simulink library "UserBlocks"  (R2014a)
settings: Solver=ode45  SolverMode=SingleTasking  StartTime=0.0  StopTime=10.0  RelTol=1e-3
values from neighbouring files (symbols this model uses):
  a = param.a    [DSC_Control_Analysis.m]    (also in DSC_Control_Analysis_Exp.m; DSC_Speed_Control_Analysis.m; EmpiricalTireCurves.m = 1.35; FFW_Fx.m = sqrt(curvature/(2*clothoidLength)))
  b = 1.15    [EmpiricalTireCurves.m]
  Cfls = Cfl    [EC_params_nissan.m]
  Crls = Crl    [EC_params_nissan.m]
  d0 = CSTR.d0    [Ext_MPCPara.m]
  freq = Fs/2*linspace(0,1,NFFT/2)    [AACplottingcode.m]    (also in If_alpha_tp_observer.m; If_alpha_tp_observer_for_c_code.m; If_alpha_tp_observer_shoreline.m)
  Iz = param.Iz    [DSC_Control_Analysis.m]    (also in DSC_Control_Analysis_Exp.m; DSC_Speed_Control_Analysis.m; EmpiricalTireCurves.m = 1300)
  K = 10    [EC_params_nissan.m]
  Ks = -10    [EC_params_nissan.m]
  Ksl = -10    [EC_params_nissan.m]
  Kt = 40000    [EC_params_nissan.m]
  Ku = -40000    [EC_params_nissan.m]
  m = 1724    [EmpiricalTireCurves.m]
  mu_s = mu_p    (= 0.6)    [EC_params_nissan.m]    (also in EmpiricalTireCurves.m = 0.55)
  Ns = 10    [EC_params_nissan.m]
  num = num+MTnum(m)    [Build_MtMuMy.m]
  q = 1    [EC_params_nissan.m]
  Taoh = CSTR.Taoh    [Ext_MPCPara.m]
  Ts = 0.002    [DSC_Control_Analysis.m]    (also in DSC_Control_Analysis_Exp.m; DSC_Speed_Control_Analysis.m; EC_params_nissan.m; Ext_MPCPara.m = SSD.Ts)
undefined symbols (not defined in the file or in its folder): acceAmp, ack, alphaFrontSteeringLimit, alphaFrontTable, bit, c, Cfl, Crl, CSTR, dden, deltaPsiDotGain, deltDist, den, denafilt, dnum, elaDotGain, filtera, filterb, frontAlphaLookup, frontForceLookup, FuelStartCalTime, FyFtable, gpsins, h, h_roll, hal_filter_den, hal_filter_num, hwx, hwy5, initAcce, initSpeed, isDriverNoise, lkparams, mapDataFull, mapMatchingParams, maxFrontForce, maxNumSegs, mdPtrs, numafilt, param, rearAlphaLookup, rfl, rfr, rrl, rrr, sglu, SIMP, simuCond, slimFxl, slimFxu, sliml, slimMll, slimMlr, slimMul, slimMur, slimu, sr, SSD, Standard, steering_limit ... (+7)
libraries: simulink x28, slrtlib x18, UserBlocks x6, slrtsoftinglib x6, MickLibBlocks x1, DriftControllerLibrary x1
(part 2 of 6)

== system UserBlocks/Diagnostic System/Filtering ==
  Residuals : Inport
  Another low-pass filter : Subsystem
      mask init:
      | %[num,den]=ellip(4,1,100,.01);
      | num=1e-4*[0.10928026599394  -0.39276857908969   0.56935540895543  -0.39276857908970   0.10928026599394];
      | den=[1  -3.96909955856226   5.90874845132499  -3.91017494417814   0.97052631831922];
  Bus Creator : BusCreator  Inputs=8
  Bus Selector : BusSelector  OutputSignals=Resistance,Motor Constant,Lsa,Rsa,yr,Gearbox Angle,Steering Angle,Current Error
  Low-pass filter : Subsystem
      mask init:
      | %[num,den]=ellip(4,1,100,.1);
      | num=1e-3*[0.23296035547458   0.49053981729288   0.64935382394602   0.49053981729287   0.23296035547457];
      | den=[1  -3.60782459052443   4.97952457348602  -3.11098657182084   0.74163873692417];
  Filtered Residuals : Outport
  wires:
  Residuals/1 -> Bus Selector/1
  Bus Selector/7 -> Bus Creator/7  "<Steering Angle>"
  Bus Selector/1 -> Bus Creator/1  "<Resistance>"
  Bus Selector/2 -> Bus Creator/2  "<Motor Constant>"
  Bus Selector/3 -> Bus Creator/3  "<Lsa>"
  Bus Selector/4 -> Bus Creator/4  "<Rsa>"
  Bus Selector/5 -> Bus Creator/5  "<yr>"
  Bus Selector/6 -> Low-pass filter/1(In1)  "<Gearbox Angle>"
  Bus Creator/1 -> Filtered Residuals/1
  Bus Selector/8 -> Another low-pass filter/1(In1)  "<Current Error>"
  Another low-pass filter/1(Out1) -> Bus Creator/8  "Filtered Current Error"
  Low-pass filter/1(Out1) -> Bus Creator/6  "Filtered Gearbox Angle"

== system UserBlocks/Diagnostic System/Isolation ==
  Boolean Residuals : Inport
  Fcn : Fcn  Expr=u[1]+2*u[2]+4*u[3]+8*u[4]+16*u[5]+32*u[6]+64*u[7]+128*u[8]+256*u[9]+512*u[10]+1024*u[11]+2048*u[12]+4096*u[13]
  Diagnosis : Outport
  wires:
  Boolean Residuals/1 -> Fcn/1
  Fcn/1 -> Diagnosis/1

== system UserBlocks/Diagnostic System/Residual Generation ==
  Steering Motors : Inport
  INS : Inport  Port=2
  Wheelspeeds : Inport  Port=3
  Current Commands : Inport  Port=4
  Handwheel : Inport  Port=5
  Roll Angle : Inport  Port=6
  Amplifier Model : Subsystem
      mask init:
      | p1_params
  Average : Gain  Gain=.5*[ 1 1]  Multiplication=Matrix(K*u)  SaturateOnIntegerOverflow=on  OutDataTypeStr=Inherit: Same as input  ParamDataTypeStr=Inherit: Same as input
  Bus Creator : BusCreator  Inputs=11
  Controller Model : Subsystem
      mask init:
      | p1_params
      | SteeringController
  Gearbox Model : Subsystem
      mask init:
      | p1_params
  Ground{,1..5} (6 alike) : Ground
  Jihan!!! : Gain  Gain=pi/180  SaturateOnIntegerOverflow=on  OutDataTypeStr=Inherit: Same as input  ParamDataTypeStr=Inherit: Same as input
  Motor Parameter Estimators : Subsystem
      mask init:
      | p1_params
      | InitMotorEstimator
  Select: Yaw Rate : Subsystem  mask{indices=1, width=6}
      mask prompts: indices "Signal indices"; width "Input width"
      mask init:
      | ic=length(indices);
      | 
      | K=zeros(ic,width);
      | 
      | for ii=1:ic,
      | 	K(ii,indices(ii))=1;
      | end
      mask Display: disp(indices)
  Terminator{,1..4} (5 alike) : Terminator
  Residuals : Outport
  wires:
  Steering Motors/1 -> Motor Parameter Estimators/1(Steering Motors), Gearbox Model/1("Steering Motors "), Controller Model/1("Steering Motors "), Amplifier Model/1("Steering Motors "), Terminator/1
  Motor Parameter Estimators/1(Resistances) -> Bus Creator/1  "Resistance"
  Motor Parameter Estimators/2(Motor Constants) -> Bus Creator/2  "Motor Constant"
  Bus Creator/1 -> Residuals/1
  Current Commands/1 -> Motor Parameter Estimators/2(Current Commands), Amplifier Model/2(Current Commands), Terminator2/1
  Select: Yaw Rate/1(Out1) -> Terminator1/1
  INS/1 -> Select: Yaw Rate/1(In1)
  Average/1 -> Terminator3/1
  Wheelspeeds/1 -> Average/1
  Gearbox Model/1(A) -> Bus Creator/9  "Gearbox Angle"
  Controller Model/1(B) -> Bus Creator/10  "Steering Angle"
  Handwheel/1 -> Controller Model/2(Handwheel)
  Amplifier Model/1(B) -> Bus Creator/11  "Current Error"
  Roll Angle/1 -> Jihan!!!/1
  Jihan!!!/1 -> Terminator4/1
  Ground/1 -> Bus Creator/3  "Yaw Rate A"
  Ground1/1 -> Bus Creator/4  "Yaw Rate B"
  Ground2/1 -> Bus Creator/5  "Yaw Rate C"
  Ground3/1 -> Bus Creator/6  "Lsa"
  Ground4/1 -> Bus Creator/7  "Rsa"
  Ground5/1 -> Bus Creator/8  "yr"

== system UserBlocks/EnvEnv Connection/Ackermann Correction ==
  Ackermann Angle : Inport
  left ackermann ideal correction angle : Fcn  Expr=u/(1-u*ack*param.tw/2/(param.a+param.b))
  right ackermann ideal correction angle : Fcn  Expr=u/(1+u*ack*param.tw/2/(param.a+param.b))
  L Steer Angle : Outport
  R Steer Angle : Outport  Port=2
  wires:
  Ackermann Angle/1 -> right ackermann ideal correction angle/1, left ackermann ideal correction angle/1
  right ackermann ideal correction angle/1 -> R Steer Angle/1
  left ackermann ideal correction angle/1 -> L Steer Angle/1

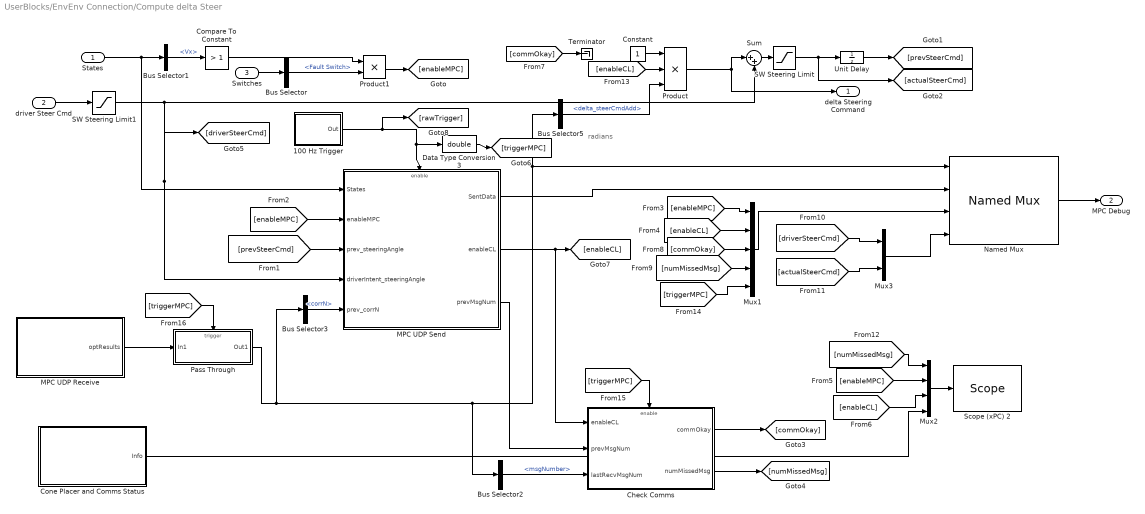
== system UserBlocks/EnvEnv Connection/Compute delta Steer ==
  note: radians
  States : Inport
  driver Steer Cmd : Inport  Port=2
  Switches : Inport  Port=3
  100 Hz Trigger : Subsystem
  Bus Selector : BusSelector  OutputSignals=Fault Switch
  Bus Selector1 : BusSelector  OutputSignals=Vx
  Bus Selector2 : BusSelector  OutputSignals=msgNumber
  Bus Selector3 : BusSelector  OutputSignals=corrN
  Bus Selector5 : BusSelector  OutputSignals=delta_steerCmdAdd
  Check Comms : Subsystem  TreatAsAtomicUnit=on
  Compare To Constant : simulink/Logic and Bit Operations/Compare To Constant  relop=>  const=1  OutDataTypeStr=uint8  ZeroCross=off
  Cone Placer and Comms Status : Subsystem
  Constant : Constant
  Data Type Conversion3 : DataTypeConversion  OutDataTypeStr=double
  MPC UDP Receive : Subsystem
  MPC UDP Send : Subsystem
  Mux1 : Mux  Inputs=5
  Mux2 : Mux
  Mux3 : Mux  Inputs=2
  Named Mux : UserBlocks/MPC CAN Connection/Named Mux  fname=datadescEnvEnv
  Pass Through : Subsystem  TreatAsAtomicUnit=on
  Product : Product  Inputs=3  RndMeth=Zero
  Product1 : Product  RndMeth=Zero
  SW Steering Limit : Saturate  UpperLimit=steering_limit*pi/180  LowerLimit=-steering_limit*pi/180
  SW Steering Limit1 : Saturate  UpperLimit=steering_limit*pi/180  LowerLimit=-steering_limit*pi/180
  Scope (xPC) 2 : slrtlib/Displays and Logging/Scope   scopeno=2  scopetype=Target  autostart=on  viewmode=Numerical  formatstr="' Missed Msgs:   %6.0f, EnableMPC:    %1.0f, EnableCL:     %1.0f, Bumper E Pos [m]:    %4.2f, Bumper N Pos [m]:    %4.2f, Num Laptop Msgs: %5.0f, Num Veh Msgs:    %5.0f'"  grid=on  ylimits=[0,0]  nosamples=round(1/Ts)/20  noprepostsamples=0  interleave=1  triggermode=FreeRun  triggersignal=1  trigsignalfromport=off  triggerlevel=0.0  triggerslope=Either  triggerscope=1  triggersample=0  filename=data.dat  mode=Lazy  writesize=512  autorestart=off  dynamicfilemode=off  maxwritefilesize=512*1024^2
  Sum : Sum  Inputs=|++
  Terminator : Terminator
  Unit Delay : UnitDelay  SampleTime=-1
  delta Steering Command : Outport
  MPC Debug : Outport  Port=2
  wires:
  Cone Placer and Comms Status/1(Info) -> Mux2/4
  [numMissedMsg] -> Mux2/1
  [enableCL] -> Mux2/3
  [enableMPC] -> Mux2/2
  Mux2/1 -> Scope (xPC) 2/1
  Bus Selector3/1 -> MPC UDP Send/5(prev_corrN)  "<corrN>"
  [triggerMPC] -> Pass Through/Trigger
  MPC UDP Receive/1(optResults) -> Pass Through/1(In1)
  MPC UDP Send/3(prevMsgNum) -> Check Comms/2(prevMsgNum)
  Bus Selector2/1 -> Check Comms/3(lastRecvMsgNum)  "<msgNumber>"
  [triggerMPC] -> Check Comms/Enable
  Check Comms/2(numMissedMsg) -> [numMissedMsg]
  Check Comms/1(commOkay) -> [commOkay]
  Data Type Conversion3/1 -> [triggerMPC]
  [triggerMPC] -> Mux1/5
  Pass Through/1(Out1) -> Bus Selector3/1, Bus Selector5/1, Named Mux/1, Bus Selector2/1
  Mux1/1 -> Named Mux/3
  Constant/1 -> Product/1
  [commOkay] -> Terminator/1
  [enableCL] -> Product/2
  MPC UDP Send/2(enableCL) -> Check Comms/1(enableCL), [enableCL]
  [enableMPC] -> MPC UDP Send/2(enableMPC)
  100 Hz Trigger/1(Out) -> [rawTrigger], Data Type Conversion3/1, MPC UDP Send/Enable
  Sum/1 -> SW Steering Limit/1
  Unit Delay/1 -> [prevSteerCmd]
  SW Steering Limit/1 -> [actualSteerCmd], Unit Delay/1
  driver Steer Cmd/1 -> SW Steering Limit1/1
  [actualSteerCmd] -> Mux3/2
  [driverSteerCmd] -> Mux3/1
  Mux3/1 -> Named Mux/4
  SW Steering Limit1/1 -> [driverSteerCmd], MPC UDP Send/4(driverIntent_steeringAngle), Sum/2
  [numMissedMsg] -> Mux1/4
  [commOkay] -> Mux1/3
  Product/1 -> delta Steering Command/1, Sum/1
  [enableCL] -> Mux1/2
  [enableMPC] -> Mux1/1
  MPC UDP Send/1(SentData) -> Named Mux/2
  [prevSteerCmd] -> MPC UDP Send/3(prev_steeringAngle)
  Named Mux/1 -> MPC Debug/1
  Bus Selector5/1 -> Product/3  "<delta_steerCmdAdd>"
  Bus Selector1/1 -> Compare To Constant/1  "<Vx>"
  States/1 -> MPC UDP Send/1(States), Bus Selector1/1
  Switches/1 -> Bus Selector/1
  Bus Selector/1 -> Product1/2  "<Fault Switch>"
  Compare To Constant/1 -> Product1/1
  Product1/1 -> [enableMPC]

== system UserBlocks/EnvEnv Connection/Subsystem ==
  Handwheel : Inport
  Switches : Inport  Port=2
  Bus Selector2 : BusSelector  OutputSignals=Primary
  Bus Selector4 : BusSelector  OutputSignals=Auto-Steer Switch
  HAL-9000 : UserBlocks/Steering Controller/HAL-9000  enabled=on  maneuver=Step  amplitude=12/sr  delay=1  duration=10  startfreq=.7  endfreq=.7
  Heavy Filter : DiscreteFilter  Numerator=hal_filter_num  Denominator=hal_filter_den  SampleTime=Ts
  Nominal Filter : DiscreteFilter  Numerator=[10*2*pi*Ts]  Denominator=[1 10*2*pi*Ts-1]  SampleTime=Ts
  Steering Ratio : Gain  Gain=1/10  SaturateOnIntegerOverflow=on  OutDataTypeStr=Inherit: Same as input  ParamDataTypeStr=Inherit: Same as input
  Steering Ratio1 : Gain  Gain=1/10  SaturateOnIntegerOverflow=on  OutDataTypeStr=Inherit: Same as input  ParamDataTypeStr=Inherit: Same as input
  Sum1 : Sum  Inputs=++|
  Switch : Switch  Threshold=0.5
  Steering Output : Outport
  wires:
  Switch/1 -> Steering Output/1
  Sum1/1 -> Switch/1
  HAL-9000/1 -> Sum1/2
  Steering Ratio1/1 -> Sum1/1
  Steering Ratio/1 -> Switch/3
  Switches/1 -> Bus Selector4/1
  Bus Selector4/1 -> Switch/2, HAL-9000/1  "<Auto-Steer Switch>"
  Heavy Filter/1 -> Steering Ratio1/1
  Bus Selector2/1 -> Heavy Filter/1, Nominal Filter/1  "<Primary>"
  Nominal Filter/1 -> Steering Ratio/1
  Handwheel/1 -> Bus Selector2/1

== system UserBlocks/Envelope control with Differential drive/acc_noise_cut_filter ==
  In1 : Inport
  Butterworth Filter : DiscreteFilter  Numerator=numafilt  Denominator=denafilt  SampleTime=0.002
  Out1 : Outport
  wires:
  In1/1 -> Butterworth Filter/1
  Butterworth Filter/1 -> Out1/1

== system UserBlocks/Envelope control with Differential drive/acc_noise_cut_filter1 ==
  In1 : Inport
  Butterworth Filter : DiscreteFilter  Numerator=numafilt  Denominator=denafilt  SampleTime=0.002
  Out1 : Outport
  wires:
  Butterworth Filter/1 -> Out1/1
  In1/1 -> Butterworth Filter/1

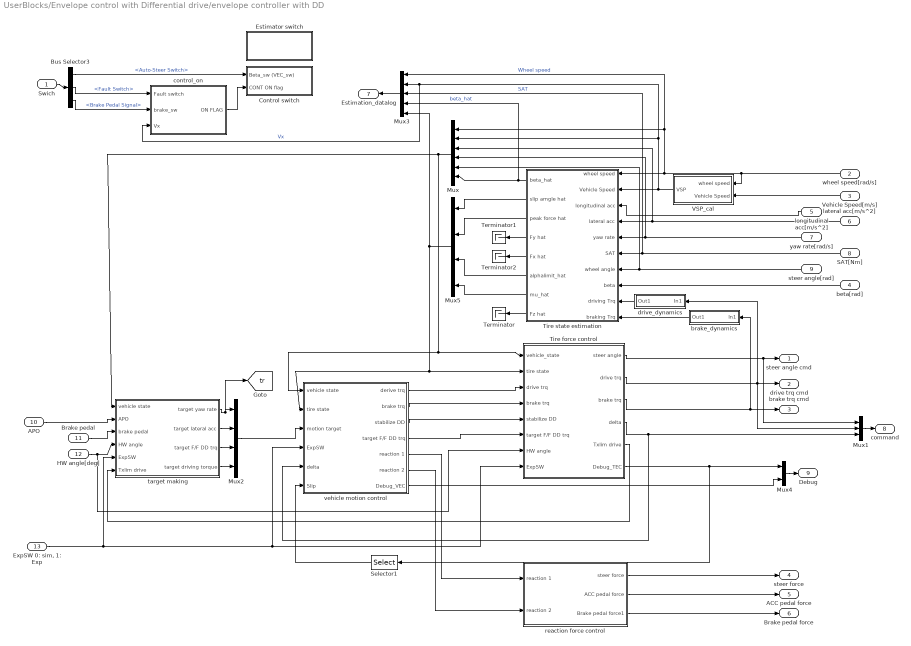
== system UserBlocks/Envelope control with Differential drive/envelope controller with DD ==
  Swich : Inport
  wheel speed[rad/s] : Inport  Port=2
  Vehicle Speed[m/s] : Inport  Port=3
  beta[rad] : Inport  Port=4
  longitudinal acc[m/s^2] : Inport  Port=5
  lateral acc[m/s^2] : Inport  Port=6
  yaw rate[rad/s] : Inport  Port=7
  SAT[Nm] : Inport  Port=8
  steer angle[rad] : Inport  Port=9
  APO : Inport  Port=10
  Brake pedal : Inport  Port=11
  HW angle[deg] : Inport  Port=12
  "ExpSW 0: sim, 1: Exp" : Inport  Port=13
  Bus Selector3 : BusSelector  OutputSignals=Auto-Steer Switch,Fault Switch,Brake Pedal Signal
  Control switch : Subsystem
  Estimator switch : Subsystem
  Mux : Mux  Inputs=6
  Mux1 : Mux  Inputs=3
  Mux2 : Mux
  Mux3 : Mux  Inputs=5
  Mux4 : Mux  Inputs=2
  Mux5 : Mux
  Selector1 : Selector  InputPortWidth=8  Indices=[5:6]
  Terminator : Terminator
  Terminator1 : Terminator
  Terminator2 : Terminator
  Tire force control : Subsystem
      mask init:
      | p1_params
      | EC_params_nissan
      | load slimmap
      | [filterb,filtera]=butter(2,0.03);
  Tire state estimation : Subsystem
      mask init:
      | p1_params
      | EC_params_nissan
  VSP_cal : Subsystem
      mask init:
      | p1_params
      | EC_params_nissan
  brake_dynamics : Subsystem
  control_on : Subsystem
  drive_dynamics : Subsystem
  reaction force control : Subsystem
  target making : Subsystem
      mask init:
      | p1_params
      | EC_params_nissan
      | % FFDDmodel_cal
      | [dnum,dden]=c2dm([1 0],[0.1 1],0.002,'tustin');
  vehicle motion control : Subsystem
      mask init:
      | p1_params
      | EC_params_nissan
      | load stableareamap.mat
  steer angle cmd : Outport
  drive trq cmd : Outport  Port=2
  brake trq cmd : Outport  Port=3
  steer force : Outport  Port=4
  ACC pedal force : Outport  Port=5
  Brake pedal force : Outport  Port=6
  Estimation_datalog : Outport  Port=7
  command : Outport  Port=8
  Debug : Outport  Port=9
  tag scope: tr=global
  wires:
  vehicle motion control/4(target F/F DD trq) -> Tire force control/6(target F/F DD trq)
  Selector1/1 -> vehicle motion control/6(Slip)
  Tire force control/5(Txlim drive) -> target making/6(Txlim drive)
  target making/4(target driving torque) -> Mux2/4
  lateral acc[m/s^2]/1 -> Mux/3, Tire state estimation/4(lateral acc)
  yaw rate[rad/s]/1 -> Mux/4, Tire state estimation/5(yaw rate)
  HW angle[deg]/1 -> target making/4(HW angle), Tire force control/7(HW angle)
  APO/1 -> target making/2(APO)
  Brake pedal/1 -> target making/3(brake pedal)
  target making/2(target lateral acc) -> Mux2/2
  target making/3(target F/F DD trq) -> Mux2/3
  Mux2/1 -> vehicle motion control/3(motion target)
  Tire force control/1(steer angle) -> steer angle cmd/1, Mux1/1
  Tire force control/2(drive trq) -> drive trq cmd/1, drive_dynamics/1(In1), Mux1/2
  Tire force control/3(brake trq) -> brake trq cmd/1, brake_dynamics/1(In1)
  vehicle motion control/1(derive trq) -> Tire force control/3("drive trq ")
  vehicle motion control/2(brake trq) -> Tire force control/4("brake trq ")
  vehicle motion control/5(reaction 1) -> reaction force control/1(reaction 1)
  vehicle motion control/6(reaction 2) -> reaction force control/2(reaction 2)
  reaction force control/1(steer force) -> steer force/1
  reaction force control/2(ACC pedal force) -> ACC pedal force/1
  reaction force control/3(Brake pedal force1) -> Brake pedal force/1
  wheel speed[rad/s]/1 -> Mux/1, Mux3/1, Tire state estimation/1(wheel speed), VSP_cal/1(wheel speed)  "Wheel speed"
  SAT[Nm]/1 -> Mux3/3, Tire state estimation/6(SAT)  "SAT"
  Tire state estimation/2(slip amgle hat) -> Mux5/1
  Tire state estimation/3(peak force hat) -> Mux5/2
  Tire state estimation/8(Fz hat) -> Terminator/1
  Mux3/1 -> Estimation_datalog/1
  vehicle motion control/3(stabilize DD) -> Tire force control/5(stabilize DD)
  Mux/1 -> vehicle motion control/1(vehicle state), Tire force control/1(vehicle_state), target making/1(vehicle state)
  Mux5/1 -> vehicle motion control/2(tire state), Tire force control/2(tire state), Mux3/5
  drive_dynamics/1(Out1) -> Tire state estimation/9(driving Trq)
  brake_dynamics/1(Out1) -> Tire state estimation/10(braking Trq)
  steer angle[rad]/1 -> Mux/5, Tire state estimation/7(wheel angle)
  Tire force control/4(delta) -> vehicle motion control/5(delta), Mux1/3
  target making/1(target yaw rate) -> Mux2/1, [tr]
  beta[rad]/1 -> Tire state estimation/8(beta)
  Tire state estimation/1(beta_hat) -> Mux/6, Mux3/4  "beta_hat"
  VSP_cal/1(VSP) -> control_on/3(Vx), Mux3/2, Mux/2, Tire state estimation/2(Vehicle Speed)  "Vx"
  Vehicle Speed[m/s]/1 -> VSP_cal/2(Vehicle Speed)
  Mux1/1 -> command/1
  Tire state estimation/4(Fy hat) -> Terminator1/1
  Tire state estimation/5(Fx hat) -> Terminator2/1
  Tire state estimation/7(mu_hat) -> Mux5/4
  Tire state estimation/6(alphalimit_hat) -> Mux5/3
  Tire force control/6(Debug_TEC) -> Selector1/1, Mux4/1
  vehicle motion control/7(Debug_VEC) -> Mux4/2
  Mux4/1 -> Debug/1
  "ExpSW 0: sim, 1: Exp"/1 -> target making/5(ExpSW), vehicle motion control/4(ExpSW), Tire force control/8(ExpSW)
  longitudinal acc[m/s^2]/1 -> Tire state estimation/3(longitudinal acc)
  control_on/1(ON FLAG) -> Control switch/2(CONT ON flag)
  Swich/1 -> Bus Selector3/1
  Bus Selector3/2 -> control_on/1(Fault switch)  "<Fault Switch>"
  Bus Selector3/3 -> control_on/2(brake_sw)  "<Brake Pedal Signal>"
  Bus Selector3/1 -> Control switch/1(Beta_sw (VEC_sw))  "<Auto-Steer Switch>"

== system UserBlocks/Envelope control with Differential drive/wheel_speed_dynamics ==
  In1 : Inport
  Butterworth Filter{,1..3} (4 alike) : DiscreteFilter  Numerator=filterb  Denominator=filtera  SampleTime=0.002
  Demux : Demux
  Mux : Mux
  rev/s to rad/s : Gain  Gain=2*pi
  ticks/sample to rev/s : Gain  Gain="1/(48*2)  *  1/Ts"
  Out1 : Outport
  wires:
  Demux/4 -> Butterworth Filter2/1
  Demux/3 -> Butterworth Filter3/1
  Demux/2 -> Butterworth Filter/1
  Demux/1 -> Butterworth Filter1/1
  Mux/1 -> Out1/1
  Butterworth Filter/1 -> Mux/1
  Butterworth Filter1/1 -> Mux/2
  Butterworth Filter2/1 -> Mux/3
  Butterworth Filter3/1 -> Mux/4
  ticks/sample to rev/s/1 -> rev/s to rad/s/1
  rev/s to rad/s/1 -> Demux/1
  In1/1 -> ticks/sample to rev/s/1

== system UserBlocks/LQACC/PIDACC ==
  Switches : Inport
  Vehicle States : Inport  Port=2
  Go Pedal1 : Inport  Port=3
  Bus Creator : BusCreator  Inputs=2
  Bus Selector : BusSelector  OutputSignals=Vx,axCG
  Bus Selector1 : BusSelector  OutputSignals=Fault Switch
  Car-Following System : Subsystem
  Demux : Demux  Outputs=3
  Discrete Filter : DiscreteFilter  Numerator=[0.006]  Denominator=[1.006 -1]  SampleTime=0.002
  MPC MTCACC : Subsystem
  PreVehicle : Subsystem
  Selection : Constant  Value=simuCond
  Subsystem : Subsystem
  Switch1 : Switch  Criteria=u2 > Threshold  Threshold=0.5
  FxCommands(N) : Outport
  PreAcce(m/s2) : Outport  Port=2
  PreSpeec(m/s) : Outport  Port=3
  epsilon : Outport  Port=4
  DesDist(m) : Outport  Port=5
  ActDist(m) : Outport  Port=6
  desAcce(m/s2) : Outport  Port=7
  distErr : Outport  Port=8
  relVEL : Outport  Port=9
  vehACCE : Outport  Port=10
  wires:
  Discrete Filter/1 -> Subsystem/1(ax), desAcce(m/s2)/1
  MPC MTCACC/2(desAcce) -> Discrete Filter/1
  Demux/3 -> vehACCE/1
  Demux/2 -> relVEL/1
  Demux/1 -> distErr/1
  Subsystem/1(Volt(V)1) -> Switch1/1
  Bus Selector/2 -> Car-Following System/4(vehAcce)  "<axCG>"
  Bus Selector/1 -> Car-Following System/3(vehSpd)  "<Vx>"
  Car-Following System/5(DesDist) -> DesDist(m)/1
  MPC MTCACC/1(epsilon) -> epsilon/1
  Car-Following System/3(actDist) -> MPC MTCACC/3(actDist), ActDist(m)/1
  Car-Following System/2(PV_acce) -> MPC MTCACC/2(PreAcce)
  Car-Following System/4(VehSpd) -> MPC MTCACC/4(vehSpd)
  PreVehicle/2(PreSpeed) -> Car-Following System/2(PVvel), PreSpeec(m/s)/1
  PreVehicle/1(PreAcce) -> Car-Following System/1(PVacce), PreAcce(m/s2)/1
  Selection/1 -> PreVehicle/1(Pattern)
  Car-Following System/1(SysOut) -> Demux/1, MPC MTCACC/1(SysOut)
  Switches/1 -> Bus Selector1/1
  Vehicle States/1 -> Bus Selector/1
  Bus Selector1/1 -> Switch1/2  "<Fault Switch>"
  Switch1/1 -> Bus Creator/1, Bus Creator/2
  Bus Creator/1 -> FxCommands(N)/1
  Go Pedal1/1 -> Switch1/3

== system UserBlocks/MPC CAN Connection/Ackermann Correction ==
  Ackermann Angle : Inport
  left ackermann ideal correction angle : Fcn  Expr=u/(1-u*ack*param.tw/2/(param.a+param.b))
  right ackermann ideal correction angle : Fcn  Expr=u/(1+u*ack*param.tw/2/(param.a+param.b))
  L Steer Angle : Outport
  R Steer Angle : Outport  Port=2
  wires:
  left ackermann ideal correction angle/1 -> L Steer Angle/1
  right ackermann ideal correction angle/1 -> R Steer Angle/1
  Ackermann Angle/1 -> left ackermann ideal correction angle/1, right ackermann ideal correction angle/1

== system UserBlocks/MPC CAN Connection/Force Feedback ==
  MPC Addition : Inport
  Feedback gain : Gain  Gain=steer_gain
  Saturation1 : Saturate  UpperLimit=current_limit  LowerLimit=-current_limit
  FFB Current : Outport
  wires:
  Feedback gain/1 -> Saturation1/1
  MPC Addition/1 -> Feedback gain/1
  Saturation1/1 -> FFB Current/1

== system UserBlocks/MPC CAN Connection/MPC CAN Receive ==
  "CAN bit-unpacking " : slrtlib/CAN/Utilities/CAN bit-unpacking   bitpatterns={ [0:15],[16:23],[24:39] }  dtypes={ 'int16' ,'int8','uint16'}
  Compare To Zero : simulink/Logic and Bit Operations/Compare To Zero  relop=>  OutDataTypeStr=uint8  ZeroCross=off
  Convert : DataTypeConversion  OutDataTypeStr=double
  Convert1 : DataTypeConversion  OutDataTypeStr=double
  Convert2 : DataTypeConversion  OutDataTypeStr=double
  Gain5 : Gain  Gain=1/10000
  Product : Product  RndMeth=Zero
  "Receive " : slrtsoftinglib/CAN-AC2-104 SJA 1000/Receive   board=1  canPort=CAN 1  range=Standard (11-bit)  ids=[501]  lengths=[8]  output=Data  inten=off  ts=0.002  ididx=[0]
  Steering Addition : Outport
  Solver Steps : Outport  Port=2
  Objective (All) : Outport  Port=3
  wires:
  "Receive "/1 -> "CAN bit-unpacking "/1
  Compare To Zero/1 -> Product/2
  Gain5/1 -> Product/1
  Convert/1 -> Gain5/1
  Convert1/1 -> Compare To Zero/1, Solver Steps/1
  "CAN bit-unpacking "/1 -> Convert/1
  "CAN bit-unpacking "/2 -> Convert1/1
  "CAN bit-unpacking "/3 -> Convert2/1
  Product/1 -> Steering Addition/1
  Convert2/1 -> Objective (All)/1

== system UserBlocks/MPC CAN Connection/MPC CAN Send ==
  Sideslip : Inport
  Yaw Rate : Inport  Port=2
  Ux : Inport  Port=3
  Steer Angle : Inport  Port=4
  Accelerator : Inport  Port=5
  Friction Est : Inport  Port=6
  Bus Selector1 : BusSelector  OutputSignals=muhat
  "CAN bit-packing " : slrtlib/CAN/Utilities/CAN bit-packing   bitpatterns={ [0:15],[16:31],[32:47],[48:55],[56:63] }
  CAN bit-packing 1 : slrtlib/CAN/Utilities/CAN bit-packing   bitpatterns={ [0:15] }
  Constant : Constant  Value=0.7
  Data Type Conversion1 : DataTypeConversion  OutDataTypeStr=uint8  RndMeth=Nearest  SaturateOnIntegerOverflow=on
  Data Type Conversion{2..4,6} (4 alike) : DataTypeConversion  OutDataTypeStr=int16  RndMeth=Nearest  SaturateOnIntegerOverflow=on
  Data Type Conversion5 : DataTypeConversion  OutDataTypeStr=int8  RndMeth=Nearest  SaturateOnIntegerOverflow=on
  Gain{,1..2,4} (4 alike) : Gain  Gain=10000
  Gain3 : Gain  Gain=100
  Rate Transition{,1..5} (6 alike) : RateTransition  OutPortSampleTimeOpt=Inherit
  "Send " : slrtsoftinglib/CAN-AC2-104 SJA 1000/Send   board=1  canPort=CAN 1  range=Standard (11-bit)  ids=[500]  sizes=[8]  output=off  ts=0.01  ididx=[0]
  Subtract : Sum  Inputs=+-
  Terminator : Terminator
  wires:
  Gain4/1 -> Data Type Conversion6/1
  Data Type Conversion6/1 -> CAN bit-packing 1/1
  Bus Selector1/1 -> Rate Transition5/1  "<muhat>"
  Rate Transition5/1 -> Gain4/1
  CAN bit-packing 1/1 -> Terminator/1
  Friction Est/1 -> Bus Selector1/1
  "CAN bit-packing "/1 -> "Send "/1
  Data Type Conversion2/1 -> "CAN bit-packing "/1
  Data Type Conversion3/1 -> "CAN bit-packing "/2
  Gain/1 -> Data Type Conversion2/1
  Gain1/1 -> Data Type Conversion3/1
  Gain2/1 -> Data Type Conversion4/1
  Data Type Conversion4/1 -> "CAN bit-packing "/3
  Data Type Conversion5/1 -> "CAN bit-packing "/4
  Rate Transition/1 -> Gain/1
  Rate Transition1/1 -> Gain1/1
  Rate Transition2/1 -> Gain2/1
  Rate Transition3/1 -> Data Type Conversion5/1
  Sideslip/1 -> Rate Transition/1
  Yaw Rate/1 -> Rate Transition1/1
  Steer Angle/1 -> Rate Transition2/1
  Ux/1 -> Rate Transition3/1
  Accelerator/1 -> Rate Transition4/1
  Data Type Conversion1/1 -> "CAN bit-packing "/5
  Gain3/1 -> Data Type Conversion1/1
  Rate Transition4/1 -> Subtract/1
  Subtract/1 -> Gain3/1
  Constant/1 -> Subtract/2

== system UserBlocks/MPC CAN Connection/Sideslip Calc ==
  Slips : Inport
  Yaw Rate : Inport  Port=2
  Ux : Inport  Port=3
  Steer Angle : Inport  Port=4
  Add : Sum  Inputs=++-
  Divide : Product  Inputs=*/
  Gain6 : Gain  Gain=a
  Prevent Divide-by-Zero : Saturate  UpperLimit=inf  LowerLimit=2
  Selector : Selector  InputPortWidth=2  Indices=[1]
  Sideslip : Outport
  wires:
  Selector/1 -> Add/2
  Gain6/1 -> Divide/1
  Divide/1 -> Add/3
  Prevent Divide-by-Zero/1 -> Divide/2
  Add/1 -> Sideslip/1
  Steer Angle/1 -> Add/1
  Slips/1 -> Selector/1
  Yaw Rate/1 -> Gain6/1
  Ux/1 -> Prevent Divide-by-Zero/1

== system UserBlocks/MPC CAN Connection/Slip angle calculation ==
  Sideslip : Inport
  Yaw Rate : Inport  Port=2
  Ux : Inport  Port=3
  Steer Angle : Inport  Port=4
  Add : Sum  Inputs=-++
  Add1 : Sum  Inputs=+-
  Divide : Product  Inputs=*/
  Divide1 : Product  Inputs=*/
  Gain1 : Gain  Gain=b
  Gain6 : Gain  Gain=a
  Prevent Divide-by-Zero : Saturate  UpperLimit=inf  LowerLimit=2
  Front Slip Angle : Outport
  Rear Slip Angle : Outport  Port=2
  wires:
  Divide1/1 -> Add1/2
  Add1/1 -> Rear Slip Angle/1
  Gain1/1 -> Divide1/1
  Ux/1 -> Prevent Divide-by-Zero/1
  Yaw Rate/1 -> Gain1/1, Gain6/1
  Sideslip/1 -> Add1/1, Add/2
  Steer Angle/1 -> Add/1
  Add/1 -> Front Slip Angle/1
  Prevent Divide-by-Zero/1 -> Divide1/2, Divide/2
  Divide/1 -> Add/3
  Gain6/1 -> Divide/1

== system UserBlocks/MPC CAN Connection/Subsystem ==
  Handwheel : Inport
  Switches : Inport  Port=2
  Bus Selector2 : BusSelector  OutputSignals=Primary
  Bus Selector4 : BusSelector  OutputSignals=Auto-Steer Switch
  HAL-9000 : UserBlocks/Steering Controller/HAL-9000  enabled=on  maneuver=Step  amplitude=12/sr  delay=1  duration=10  startfreq=.7  endfreq=.7
  Heavy Filter : DiscreteFilter  Numerator=hal_filter_num  Denominator=hal_filter_den  SampleTime=Ts
  Nominal Filter : DiscreteFilter  Numerator=[10*2*pi*Ts]  Denominator=[1 10*2*pi*Ts-1]  SampleTime=Ts
  Steering Ratio : Gain  Gain=1/10  SaturateOnIntegerOverflow=on  OutDataTypeStr=Inherit: Same as input  ParamDataTypeStr=Inherit: Same as input
  Steering Ratio1 : Gain  Gain=1/10  SaturateOnIntegerOverflow=on  OutDataTypeStr=Inherit: Same as input  ParamDataTypeStr=Inherit: Same as input
  Sum1 : Sum  Inputs=++|
  Switch : Switch  Threshold=0.5
  Steering Output : Outport
  wires:
  Handwheel/1 -> Bus Selector2/1
  Nominal Filter/1 -> Steering Ratio/1
  Bus Selector2/1 -> Nominal Filter/1, Heavy Filter/1  "<Primary>"
  Heavy Filter/1 -> Steering Ratio1/1
  Bus Selector4/1 -> HAL-9000/1, Switch/2  "<Auto-Steer Switch>"
  Switches/1 -> Bus Selector4/1
  Steering Ratio/1 -> Switch/3
  Steering Ratio1/1 -> Sum1/1
  HAL-9000/1 -> Sum1/2
  Sum1/1 -> Switch/1
  Switch/1 -> Steering Output/1

== system UserBlocks/MPCACC/PIDACC ==
  Switches : Inport
  Vehicle States : Inport  Port=2
  Go Pedal1 : Inport  Port=3
  Bus Creator : BusCreator  Inputs=2
  Bus Selector : BusSelector  OutputSignals=Vx,axCG
  Bus Selector1 : BusSelector  OutputSignals=Fault Switch
  Car-Following System : Subsystem
  Demux : Demux  Outputs=3
  Discrete Filter : DiscreteFilter  Numerator=[0.008]  Denominator=[1.008 -1]  SampleTime=0.002
  MPC MTCACC : Subsystem
  PreVehicle : UserBlocks/LQACC/PIDACC/PreVehicle
  Saturation : Saturate  UpperLimit=0.6  LowerLimit=-1
  Selection : Constant  Value=simuCond
  Subsystem : Subsystem
  Switch1 : Switch  Criteria=u2 > Threshold  Threshold=0.5
  mdPtrs : Constant  Value=mdPtrs
  FxCommands(N) : Outport
  PreAcce(m/s2) : Outport  Port=2
  PreSpeec(m/s) : Outport  Port=3
  epsilon : Outport  Port=4
  DesDist(m) : Outport  Port=5
  ActDist(m) : Outport  Port=6
  desAcce(m/s2) : Outport  Port=7
  distErr : Outport  Port=8
  relVEL : Outport  Port=9
  vehACCE : Outport  Port=10
  wires:
  Switch1/1 -> Bus Creator/2, Bus Creator/1
  Saturation/1 -> desAcce(m/s2)/1
  Go Pedal1/1 -> Switch1/3
  Bus Creator/1 -> FxCommands(N)/1
  Bus Selector1/1 -> Switch1/2  "<Fault Switch>"
  Vehicle States/1 -> Bus Selector/1
  Switches/1 -> Bus Selector1/1
  Car-Following System/1(SysOut) -> Demux/1, MPC MTCACC/1(SysOut)
  Selection/1 -> PreVehicle/1
  PreVehicle/1 -> PreAcce(m/s2)/1, Car-Following System/1(PVacce)
  PreVehicle/2 -> PreSpeec(m/s)/1, Car-Following System/2(PVvel)
  Car-Following System/4(VehSpd) -> MPC MTCACC/4(vehSpd)
  Car-Following System/2(PV_acce) -> MPC MTCACC/2(Prevel)
  Car-Following System/3(actDist) -> MPC MTCACC/3(actDist), ActDist(m)/1
  MPC MTCACC/1(epsilon) -> epsilon/1
  Car-Following System/5(DesDist) -> DesDist(m)/1
  Bus Selector/1 -> Car-Following System/3(vehSpd)  "<Vx>"
  Bus Selector/2 -> Car-Following System/4(vehAcce)  "<axCG>"
  Subsystem/1(Volt(V)1) -> Switch1/1
  Demux/1 -> distErr/1
  Demux/2 -> relVEL/1
  Demux/3 -> vehACCE/1
  MPC MTCACC/2(desAcce) -> Discrete Filter/1
  Discrete Filter/1 -> Saturation/1, Subsystem/1(ax)
  mdPtrs/1 -> MPC MTCACC/5(mdPtrs)

== system UserBlocks/Map-Matching SCACS/SCACS Map-Matching ==
  positionEast : Inport
  positionNorth : Inport  Port=2
  yawAngle : Inport  Port=3
  vx_cg : Inport  Port=4
  enable : Inport  Port=5
  initSeg : Inport  Port=6
  Bus Creator{1,4..7} (5 alike) : BusCreator  Inputs=5
  Bus Creator3 : BusCreator  Inputs=7
  Demux{1,3..4,6..7} (5 alike) : Demux  Outputs=5
  Demux5 : Demux  Outputs=7
  Mux1 : Mux
  Mux2 : Mux  Inputs=2
  S-Function : S-Function  FunctionName=match_scacs  Parameters=0.005,30,0.9,10  EnableBusSupport=off
  matchOut : Outport
  currentOut : Outport  Port=2
  nextOut : Outport  Port=3
  twoOut : Outport  Port=4
  debugOut : Outport  Port=5
  thrOut : Outport  Port=6
  wires:
  initSeg/1 -> Mux2/2
  enable/1 -> Mux2/1  "enable"
  Mux2/1 -> S-Function/2
  vx_cg/1 -> Mux1/4
  Demux4/5 -> Bus Creator5/5  "totalDistance"
  Demux4/4 -> Bus Creator5/4  "enable"
  S-Function/4 -> Demux6/1  "twoOut"
  Demux6/5 -> Bus Creator6/5  "twoEndCurvature"
  Demux3/5 -> Bus Creator4/5  "nextEndCurvature"
  Demux5/7 -> Bus Creator3/7  "currEndCurvature"
  Bus Creator7/1 -> matchOut/1
  Demux7/5 -> Bus Creator7/5  "dst2end"
  Demux7/4 -> Bus Creator7/4  "finalSeg"
  Demux7/3 -> Bus Creator7/3  "curvature"
  Demux7/2 -> Bus Creator7/2  "deltaPsi"
  Demux7/1 -> Bus Creator7/1  "latError"
  S-Function/1 -> Demux7/1  "matchOut"
  S-Function/3 -> Demux3/1  "nextOut"
  S-Function/2 -> Demux5/1  "currentOut"
  S-Function/5 -> Demux4/1  "debugOut"
  Mux1/1 -> S-Function/1
  Demux5/1 -> Bus Creator3/1  "currCrvNum"
  Demux5/2 -> Bus Creator3/2  "currSegType"
  Demux5/3 -> Bus Creator3/3  "currSegLength"
  Demux5/4 -> Bus Creator3/4  "currSegProg"
  Demux3/1 -> Bus Creator4/1  "nextCrvNum"
  Demux3/2 -> Bus Creator4/2  "nextSegType"
  Demux3/3 -> Bus Creator4/3  "nextSegLength"
  Demux3/4 -> Bus Creator4/4  "nextStartCurvature"
  Demux4/1 -> Bus Creator5/1  "numIterations"
  Demux4/2 -> Bus Creator5/2  "wasLimit"
  Demux4/3 -> Bus Creator5/3  "residualError"
  Bus Creator3/1 -> currentOut/1
  Bus Creator4/1 -> nextOut/1
  Bus Creator5/1 -> debugOut/1
  positionEast/1 -> Mux1/1
  positionNorth/1 -> Mux1/2
  yawAngle/1 -> Mux1/3
  Demux5/5 -> Bus Creator3/5  "distToNxtSeg"
  Demux5/6 -> Bus Creator3/6  "currStartCurvature"
  Demux6/1 -> Bus Creator6/1  "twoCrvNum"
  Demux6/2 -> Bus Creator6/2  "twoSegType"
  Demux6/3 -> Bus Creator6/3  "twoSegLength"
  Demux6/4 -> Bus Creator6/4  "twoStartCurvature"
  Bus Creator6/1 -> twoOut/1
  Bus Creator1/1 -> thrOut/1
  Demux1/4 -> Bus Creator1/4  "thrStartCurvature"
  Demux1/3 -> Bus Creator1/3  "thrSegLength"
  Demux1/2 -> Bus Creator1/2  "thrSegType"
  Demux1/1 -> Bus Creator1/1  "thrCrvNum"
  Demux1/5 -> Bus Creator1/5  "thrEndCurvature"
  S-Function/6 -> Demux1/1  "thrOut"

== system UserBlocks/Offline Estimation/Data Extractor ==
  Steering Motors : Inport
  INS : Inport  Port=2
  Wheelspeeds : Inport  Port=3
  Current Commands : Inport  Port=4
  Butterworth Filter : DiscreteFilter  Numerator=filterb  Denominator=filtera  SampleTime=Ts
  Motor Current Fixup Due to Voltage Limitation : Subsystem
      mask init:
      | p1_params
      | nissan_steer_lookup_data
  Mux : Mux  Inputs=2
  Select: Left Motor Angle : Subsystem  mask{indices=1, width=8}
      mask prompts: indices "Signal indices"; width "Input width"
      mask init:
      | ic=length(indices);
      | 
      | K=zeros(ic,width);
      | 
      | for ii=1:ic,
      | 	K(ii,indices(ii))=1;
      | end
      mask Display: disp(indices)
  Select: Right Motor Angle : Subsystem  mask{indices=2, width=8}
      mask prompts: indices "Signal indices"; width "Input width"
      mask init:
      | ic=length(indices);
      | 
      | K=zeros(ic,width);
      | 
      | for ii=1:ic,
      | 	K(ii,indices(ii))=1;
      | end
      mask Display: disp(indices)
  Select: Yaw Rate : Subsystem  mask{indices=1, width=6}
      mask prompts: indices "Signal indices"; width "Input width"
      mask init:
      | ic=length(indices);
      | 
      | K=zeros(ic,width);
      | 
      | for ii=1:ic,
      | 	K(ii,indices(ii))=1;
      | end
      mask Display: disp(indices)
  Steering Geometry & Gearbox Correction : Subsystem
      mask init:
      | p1_params
      | nissan_steer_lookup_data
  Sum4 : Sum  Inputs=|++
  Yaw Gyro Bias : Constant  Value=gpsins.yaw_rate_bias
  average together : Gain  Gain=[0.5 0.5]  Multiplication=Matrix(K*u)
  rev/s to m/s : Gain  Gain=[param.fl.r ; param.fr.r]*2*pi
  ticks/sample to rev/s : Gain  Gain="1/(48*2)  *  1/Ts"
  Steer Angles : Outport
  Motor Currents : Outport  Port=2
  Yaw Rate : Outport  Port=3
  Velocity : Outport  Port=4
  wires:
  INS/1 -> Select: Yaw Rate/1(In1)
  Steering Motors/1 -> Select: Left Motor Angle/1(In1), Select: Right Motor Angle/1(In1)
  Select: Left Motor Angle/1(Out1) -> Mux/1
  Select: Right Motor Angle/1(Out1) -> Mux/2
  Mux/1 -> Steering Geometry & Gearbox Correction/1(Motor Angles), Motor Current Fixup Due to Voltage Limitation/1(Motor Angles)
  Steering Geometry & Gearbox Correction/1(Steer Angles) -> Steer Angles/1
  Select: Yaw Rate/1(Out1) -> Sum4/1
  Sum4/1 -> Yaw Rate/1
  Yaw Gyro Bias/1 -> Sum4/2
  Wheelspeeds/1 -> ticks/sample to rev/s/1
  ticks/sample to rev/s/1 -> rev/s to m/s/1
  Butterworth Filter/1 -> Velocity/1
  rev/s to m/s/1 -> average together/1
  average together/1 -> Butterworth Filter/1
  Motor Current Fixup Due to Voltage Limitation/1(Motor Currents) -> Motor Currents/1
  Current Commands/1 -> Motor Current Fixup Due to Voltage Limitation/2(Current Commands)

== system UserBlocks/Offline Estimation/Fault Maker ==
  Unfaulted : Inport
  Faulted : Outport
  wires:
  Unfaulted/1 -> Faulted/1

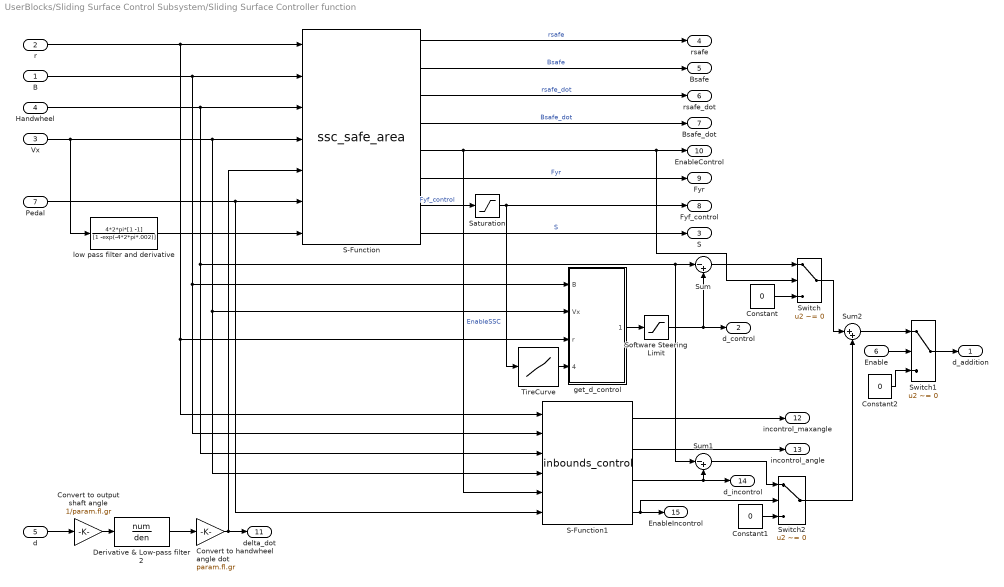
== system UserBlocks/Sliding Surface Control Subsystem/Sliding Surface Controller function ==
  B : Inport
  r : Inport  Port=2
  Vx : Inport  Port=3
  Handwheel : Inport  Port=4
  d : Inport  Port=5
  Enable : Inport  Port=6
  Pedal : Inport  Port=7
  Constant : Constant  Value=0
  Constant1 : Constant  Value=0
  Constant2 : Constant  Value=0
  Convert to handwheel angle dot : Gain  Gain=param.fl.gr  SaturateOnIntegerOverflow=on  OutDataTypeStr=Inherit: Same as input  ParamDataTypeStr=Inherit: Same as input
  Convert to output shaft angle : Gain  Gain=1/param.fl.gr  SaturateOnIntegerOverflow=on  OutDataTypeStr=Inherit: Same as input  ParamDataTypeStr=Inherit: Same as input
  Derivative & Low-pass filter 2 : DiscreteFilter  Numerator=num  Denominator=den  SampleTime=Ts
  S-Function : S-Function  FunctionName=ssc_safe_area  Parameters=a, b, CalphaF, CalphaR, Fzf, Fzr, mu, mu_s, m, Iz, bsafe_const, msafe_const, bsafe_slope, q_SSC, Kcontrol_SSC  EnableBusSupport=off
  S-Function1 : S-Function  FunctionName=inbounds_control  Parameters=a, b, CalphaF, CalphaR, Fzf, Fzr, mu, mu_s  EnableBusSupport=off
  Saturation : Saturate  UpperLimit=maxFrontForce  LowerLimit=-maxFrontForce
  Software Steering Limit : Saturate  UpperLimit=steering_limit*pi/180  LowerLimit=-steering_limit*pi/180
  Sum : Sum  Inputs=|-+
  Sum1 : Sum  Inputs=|-+
  Sum2 : Sum  Inputs=|++
  Switch : Switch  Criteria=u2 ~= 0
  Switch1 : Switch  Criteria=u2 ~= 0
  Switch2 : Switch  Criteria=u2 ~= 0
  TireCurve : Lookup  InputValues=frontForceLookup  Table=frontAlphaLookup
  get_d_control : Subsystem
  low pass filter and derivative : DiscreteTransferFcn  Numerator=4*2*pi*[1 -1]  Denominator=[1 -exp(-4*2*pi*.002)]  SampleTime=.002
  d_addition : Outport
  d_control : Outport  Port=2
  S : Outport  Port=3
  rsafe : Outport  Port=4
  Bsafe : Outport  Port=5
  rsafe_dot : Outport  Port=6
  Bsafe_dot : Outport  Port=7
  Fyf_control : Outport  Port=8
  Fyr : Outport  Port=9
  EnableControl : Outport  Port=10
  delta_dot : Outport  Port=11
  incontrol_maxangle : Outport  Port=12
  incontrol_angle : Outport  Port=13
  d_incontrol : Outport  Port=14
  EnableIncontrol : Outport  Port=15
  wires:
  Sum2/1 -> Switch1/1
  Switch2/1 -> Sum2/2
  Switch/1 -> Sum2/1
  Constant1/1 -> Switch2/3
  Sum1/1 -> Switch2/1
  S-Function1/4 -> Switch2/2, EnableIncontrol/1
  S-Function1/3 -> Sum1/2, d_incontrol/1
  S-Function1/2 -> incontrol_angle/1
  S-Function1/1 -> incontrol_maxangle/1
  Switch1/1 -> d_addition/1
  Enable/1 -> Switch1/2
  Vx/1 -> low pass filter and derivative/1, S-Function1/4, get_d_control/2(Vx), S-Function/4
  low pass filter and derivative/1 -> S-Function/7
  Pedal/1 -> S-Function1/6, S-Function/6
  Software Steering Limit/1 -> Sum/2, d_control/1
  Handwheel/1 -> Sum1/1, Sum/1, S-Function1/3, S-Function/3
  B/1 -> S-Function1/2, get_d_control/1(B), S-Function/2
  r/1 -> S-Function1/1, get_d_control/3(r), S-Function/1
  TireCurve/1 -> get_d_control/4(alphaFcontrol)
  get_d_control/1(d_control) -> Software Steering Limit/1
  Sum/1 -> Switch/1
  Constant/1 -> Switch/3
  Convert to output shaft angle/1 -> Derivative & Low-pass filter 2/1
  Derivative & Low-pass filter 2/1 -> Convert to handwheel angle dot/1
  Convert to handwheel angle dot/1 -> S-Function/5, delta_dot/1
  S-Function/1 -> rsafe/1  "rsafe"
  S-Function/2 -> Bsafe/1  "Bsafe"
  S-Function/3 -> rsafe_dot/1  "rsafe_dot"
  S-Function/4 -> Bsafe_dot/1  "Bsafe_dot"
  S-Function/5 -> S-Function1/5, EnableControl/1, Switch/2  "EnableSSC"
  S-Function/7 -> Saturation/1  "Fyf_control"
  S-Function/8 -> S/1  "S"
  S-Function/6 -> Fyr/1  "Fyr"
  Saturation/1 -> TireCurve/1, Fyf_control/1
  d/1 -> Convert to output shaft angle/1
  Constant2/1 -> Switch1/3

== system UserBlocks/Sliding Surface Control Subsystem v1/Sliding Surface Controller function ==
  B : Inport
  r : Inport  Port=2
  Vx : Inport  Port=3
  Enable : Inport  Port=4
  Handwheel : Inport  Port=5
  d : Inport  Port=6
  Constant1 : Constant  Value=0
  Kcontrol : Subsystem  AncestorBlock=UserBlocks/Sliding Surface Control Subsystem/Sliding Surface Controller function/getFyr
  Product : Product  RndMeth=Zero
  S-Function : S-Function  FunctionName=discrete_bike_nonlinear  Parameters=a, b, CalphaF, CalphaR, Fzf, Fzr, mu, mu_s, T, m, Iz  EnableBusSupport=off
  Software Steering Limit : Saturate  UpperLimit=steering_limit*pi/180  LowerLimit=-steering_limit*pi/180
  Sum : Sum  Inputs=|-+
  Switch : Switch  Threshold=Vx_threshold
  Terminator : Terminator
  TireCurve : Lookup  InputValues=frontForceLookup
  getFyf_control : Subsystem
  getFyr : Subsystem
  getSurface_S : Subsystem
  get_d_control : Subsystem
  d_addition : Outport
  d_control : Outport  Port=2
  S : Outport  Port=3
  rnom : Outport  Port=4
  Bnom : Outport  Port=5
  rnom_dot : Outport  Port=6
  Bnom_dot : Outport  Port=7
  Fyf_control : Outport  Port=8
  Fyr : Outport  Port=9
  EnableControl : Outport  Port=10
  K_control : Outport  Port=11
  wires:
  Sum/1 -> Product/2
  Enable/1 -> EnableControl/1, Product/1
  getFyr/1(Fyr) -> Fyr/1, getFyf_control/3(Fyr)
  get_d_control/1(d_control) -> Software Steering Limit/1
  TireCurve/1 -> get_d_control/4(alphaFcontrol)
  getSurface_S/1(Surface_S) -> S/1, getFyf_control/6(Surface_S)
  getFyf_control/1(Fyfcontrol) -> TireCurve/1, Fyf_control/1
  S-Function/1 -> Bnom/1, getSurface_S/3(Bnom)  "Bnom"
  r/1 -> getFyr/3(r), getSurface_S/2(r), get_d_control/3(r), getFyf_control/1(r)
  B/1 -> get_d_control/1(B), getSurface_S/1(B), getFyr/1(B)
  Handwheel/1 -> Sum/1, S-Function/2
  Vx/1 -> get_d_control/2(Vx), getFyf_control/2(Vx), Switch/2, S-Function/1, getFyr/2(Vx), Kcontrol/1(Vx)
  S-Function/3 -> getFyf_control/5(Bnomdot), Bnom_dot/1  "bnom_dot"
  Software Steering Limit/1 -> d_control/1, Sum/2
  Product/1 -> Switch/1
  Switch/1 -> d_addition/1
  Constant1/1 -> Switch/3
  d/1 -> Terminator/1
  S-Function/2 -> getSurface_S/4(rnom), rnom/1  "rnom"
  S-Function/4 -> rnom_dot/1, getFyf_control/4(rnomdot)  "rnom_dot"
  Kcontrol/1(Kcontrol) -> getFyf_control/7(Kcontrol), K_control/1

== system UserBlocks/Steering Controller/Ackermann Correction ==
  Ackermann Angle : Inport
  left ackermann ideal correction angle : Fcn  Expr=u/(1-u*ack*param.tw/2/(param.a+param.b))
  right ackermann ideal correction angle : Fcn  Expr=u/(1+u*ack*param.tw/2/(param.a+param.b))
  L Steer Angle : Outport
  R Steer Angle : Outport  Port=2
  wires:
  left ackermann ideal correction angle/1 -> L Steer Angle/1
  right ackermann ideal correction angle/1 -> R Steer Angle/1
  Ackermann Angle/1 -> left ackermann ideal correction angle/1, right ackermann ideal correction angle/1

== system UserBlocks/Steering Controller/HAL-9000 ==
  Trigger : Inport
  Amplitude : Constant  Value=amplitude*sr*pi/180
  Chirp Signal : Subsystem  mask(chirp){f1=startfreq, T=duration, f2=endfreq, VectorParams1D=on}
      mask prompts: f1 "Initial frequency (Hz):"; T "Target time (secs):"; f2 "Frequency at target time (Hz):"; VectorParams1D "Interpret vectors parameters as 1-D"
      mask help: Output a linear chirp signal (sine wave whose frequency varies linearly with time).
      mask init:
      | blkName = gcb;
      | t=[0:.1:5];
      | set_param([blkName '/targetTime'], 'VectorParams1D', VectorParams1D);
      | set_param([blkName '/initialFreq'], 'VectorParams1D', VectorParams1D);
      | set_param([blkName '/deltaFreq'], 'VectorParams1D', VectorParams1D);
      mask Help: The chirp signal has linearly increasing frequency with time.  This block can be used for spectral analysis of nonlinear systems.
      mask Display: plot(t,sin(t.*t))
  Clock : Clock
  Delay : Constant  Value=delay
  Double chirp : Subsystem
  Double-step : Subsystem
      mask Display: plot([0 1 1 2 2 3 3 4 4 5],[0 0 1 1 0 0 -1 -1 0 0])
  Enable : Constant  Value=enabled
  Latch : Subsystem  TreatAsAtomicUnit=on
  Maneuver : Constant  Value=maneuver
  Multiport Switch : MultiPortSwitch  Inputs=5
  Product : Product  Inputs=3  SaturateOnIntegerOverflow=on  OutDataTypeStr=Inherit: Same as first input
  Product1 : Product  SaturateOnIntegerOverflow=on  OutDataTypeStr=Inherit: Same as first input
  Ramp : Subsystem
      mask Display: plot([0 3 7 10],[1 1 8 8])
  Step : Subsystem
      mask Display: plot([0 5 5 10],[1 1 8 8])
  Sum : Sum  Inputs=|++
  Offset : Outport
  wires:
  Clock/1 -> Latch/1(In1)
  Product1/1 -> Product/1, Latch/Trigger
  Product/1 -> Offset/1
  Multiport Switch/1 -> Product/2
  Amplitude/1 -> Product/3
  Step/1(Out) -> Multiport Switch/2
  Maneuver/1 -> Multiport Switch/1
  Sum/1 -> Step/1(Start Time), Ramp/1(Start Time), Chirp Signal/1(Start Time), Double-step/1(Start Time), Double chirp/1(In1)
  Ramp/1(Out1) -> Multiport Switch/3
  Chirp Signal/1(Out2) -> Multiport Switch/4
  Latch/1(Out1) -> Sum/1
  Delay/1 -> Sum/2
  Trigger/1 -> Product1/1
  Enable/1 -> Product1/2
  Double-step/1(Out) -> Multiport Switch/5
  Double chirp/1(Out1) -> Multiport Switch/6

== system UserBlocks/TTS Steering Control/Ackermann Correction ==
  Ackermann Angle : Inport
  left ackermann ideal correction angle : Fcn  Expr=u/(1-u*ack*param.tw/2/(param.a+param.b))
  right ackermann ideal correction angle : Fcn  Expr=u/(1+u*ack*param.tw/2/(param.a+param.b))
  L Steer Angle : Outport
  R Steer Angle : Outport  Port=2
  wires:
  Ackermann Angle/1 -> right ackermann ideal correction angle/1, left ackermann ideal correction angle/1
  right ackermann ideal correction angle/1 -> R Steer Angle/1
  left ackermann ideal correction angle/1 -> L Steer Angle/1

== system UserBlocks/TTS Steering Control/Compute Steering Along Path ==
  States : Inport
  Switches : Inport  Port=2
  Bus Creator : BusCreator  Inputs=2
  Bus Creator1 : BusCreator  Inputs=2
  Bus Creator2 : BusCreator
  FFWsteeringNonlinear : Subsystem
      mask init:
      | TTSsteeringParams
  Feedback Steering Edit : Subsystem  TreatAsAtomicUnit=on
      mask init:
      | TTSsteeringParams
  Force2delta : Subsystem
      mask init:
      | TTSsteeringParams
  Limited Steering : Subsystem  TreatAsAtomicUnit=on
      mask init:
      | TTSsteeringParams
  Named Mux : DriftControllerLibrary/Driftkeeping/Driftkeeping Subsystem/Named Mux  fname=datadescTTSsteering
  StaticMap : Subsystem
      mask init:
      | TTSsteeringParams
  Terminator : Terminator
  desiredSpeed Dynamic Maps : Subsystem
      mask init:
      | TTSsteeringParams
  delta (rad) : Outport
  debug : Outport  Port=2
  wires:
  Switches/1 -> Terminator/1
  Bus Creator2/1 -> Named Mux/2
  Force2delta/2(FFWsteeringSSsignals) -> Bus Creator2/3
  Named Mux/1 -> debug/1
  Bus Creator1/1 -> Named Mux/3
  Limited Steering/1(delta Command regulated) -> Bus Creator2/1, delta (rad)/1
  Force2delta/1(deltaSteering) -> Limited Steering/2(delta Command)
  desiredSpeed Dynamic Maps/1(UxDesired) -> Bus Creator1/1
  desiredSpeed Dynamic Maps/2(AxDesired) -> Bus Creator1/2, FFWsteeringNonlinear/3(axDesired)
  StaticMap/2(mapMatch) -> Named Mux/1, Feedback Steering Edit/1(SCACS), Force2delta/4(SCACS), FFWsteeringNonlinear/1(SCACS), desiredSpeed Dynamic Maps/2(SCACS)
  StaticMap/1(map) -> desiredSpeed Dynamic Maps/1(Map)
  Bus Creator/1 -> Bus Creator2/4, Force2delta/3(simValues)
  FFWsteeringNonlinear/3(rSim) -> Bus Creator/2  "rSim"
  FFWsteeringNonlinear/2(UySim) -> Bus Creator/1  "UySim"
  FFWsteeringNonlinear/1(FFWfrontForce) -> Force2delta/1(FFWfrontBus)  "outputFFWss"
  Feedback Steering Edit/1(deltaPsiDotFB) -> Bus Creator2/2
  Feedback Steering Edit/2(steeringFBforce) -> Force2delta/2(FBsteeringForce)
  States/1 -> FFWsteeringNonlinear/2(States), Feedback Steering Edit/2(States), Limited Steering/1(States), Force2delta/5(States), StaticMap/1(States)

== system UserBlocks/TTS Steering Control/Subsystem ==
  Handwheel : Inport
  Switches : Inport  Port=2
  Bus Selector2 : BusSelector  OutputSignals=Primary
  Bus Selector4 : BusSelector  OutputSignals=Auto-Steer Switch
  HAL-9000 : UserBlocks/Steering Controller/HAL-9000  enabled=on  maneuver=Step  amplitude=12/sr  delay=1  duration=10  startfreq=.7  endfreq=.7
  Heavy Filter : DiscreteFilter  Numerator=hal_filter_num  Denominator=hal_filter_den  SampleTime=Ts
  Nominal Filter : DiscreteFilter  Numerator=[10*2*pi*Ts]  Denominator=[1 10*2*pi*Ts-1]  SampleTime=Ts
  Steering Ratio : Gain  Gain=1/10  SaturateOnIntegerOverflow=on  OutDataTypeStr=Inherit: Same as input  ParamDataTypeStr=Inherit: Same as input
  Steering Ratio1 : Gain  Gain=1/10  SaturateOnIntegerOverflow=on  OutDataTypeStr=Inherit: Same as input  ParamDataTypeStr=Inherit: Same as input
  Sum1 : Sum  Inputs=++|
  Switch : Switch  Threshold=0.5
  Steering Output : Outport
  wires:
  Switch/1 -> Steering Output/1
  Sum1/1 -> Switch/1
  HAL-9000/1 -> Sum1/2
  Steering Ratio1/1 -> Sum1/1
  Steering Ratio/1 -> Switch/3
  Switches/1 -> Bus Selector4/1
  Bus Selector4/1 -> Switch/2, HAL-9000/1  "<Auto-Steer Switch>"
  Heavy Filter/1 -> Steering Ratio1/1
  Bus Selector2/1 -> Heavy Filter/1, Nominal Filter/1  "<Primary>"
  Nominal Filter/1 -> Steering Ratio/1
  Handwheel/1 -> Bus Selector2/1

== system UserBlocks/Cruise Control/Enable Logic/Delay ==
  In : Inport
  Unit Delay{,1..4} (5 alike) : UnitDelay  SampleTime=Ts
  Out : Outport
  wires:
  In/1 -> Unit Delay/1
  Unit Delay/1 -> Unit Delay1/1
  Unit Delay1/1 -> Unit Delay2/1
  Unit Delay2/1 -> Unit Delay3/1
  Unit Delay3/1 -> Unit Delay4/1
  Unit Delay4/1 -> Out/1

== system UserBlocks/Cruise Control/Enable Logic/Latch1 ==
  In1 : Inport
  Trigger : TriggerPort
  Out1 : Outport  InitialOutput=0
  wires:
  In1/1 -> Out1/1
